simulink model "PartA_2"  (R2016b)
settings: Solver=FixedStepAuto  StartTime=0.0  StopTime=10.0  FixedStep=0.001  RelTol=1e-3
undefined symbols (not defined in the file or in its folder): alpha
settings Model: Creator=deepika  LastModifiedBy=deepika

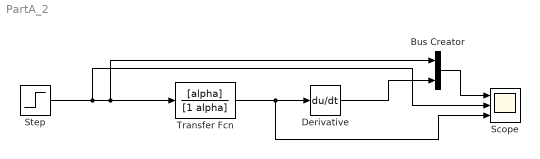
== system PartA_2 ==
  Bus Creator : BusCreator  Inputs=2
  Derivative : Derivative
  Scope : Scope  NumInputPorts=3
  Step : Step  SampleTime=0
  Transfer Fcn : TransferFcn  Numerator=[alpha]  Denominator=[1 alpha]
  wires:
  Step/1 -> Scope/2, Bus Creator/1, Transfer Fcn/1
  Transfer Fcn/1 -> Scope/3, Derivative/1
  Derivative/1 -> Bus Creator/2
  Bus Creator/1 -> Scope/1
